simulink model "iface"  (R2018b)
settings: Solver=FixedStepDiscrete  StartTime=0.0  StopTime=10.0  RelTol=1e-3
settings Model: Creator=matlab  LastModifiedBy=matlab

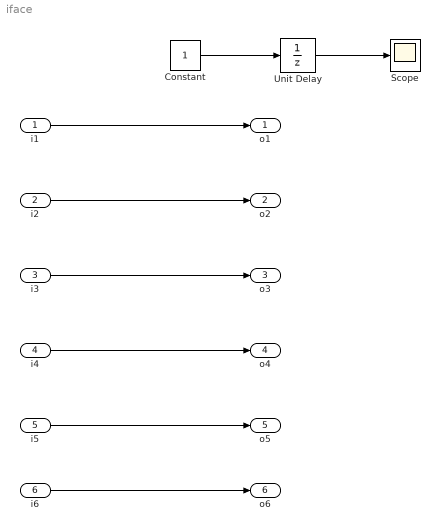
== system iface ==
  i1 : Inport  OutDataTypeStr=Enum: BoolSimulinkIntEnumType  PortDimensions=2
  i2 : Inport  Port=2  OutDataTypeStr=Enum: BoolUInt8Enum  PortDimensions=2
  i3 : Inport  Port=3  OutDataTypeStr=Enum: BoolUInt16Enum  PortDimensions=2
  i4 : Inport  Port=4  OutDataTypeStr=Enum: BoolInt8Enum  PortDimensions=2
  i5 : Inport  Port=5  OutDataTypeStr=Enum: BoolInt16Enum  PortDimensions=2
  i6 : Inport  Port=6  OutDataTypeStr=Enum: BoolInt32Enum  PortDimensions=2
  Constant : Constant
  Scope : Scope
  Unit Delay : UnitDelay  SampleTime=-1
  o1 : Outport  OutDataTypeStr=Enum: BoolSimulinkIntEnumType  PortDimensions=2
  o2 : Outport  Port=2  OutDataTypeStr=Enum: BoolUInt8Enum  PortDimensions=2
  o3 : Outport  Port=3  OutDataTypeStr=Enum: BoolUInt16Enum  PortDimensions=2
  o4 : Outport  Port=4  OutDataTypeStr=Enum: BoolInt8Enum  PortDimensions=2
  o5 : Outport  Port=5  OutDataTypeStr=Enum: BoolInt16Enum  PortDimensions=2
  o6 : Outport  Port=6  OutDataTypeStr=Enum: BoolInt32Enum  PortDimensions=2
  wires:
  i3/1 -> o3/1
  i2/1 -> o2/1
  i5/1 -> o5/1
  i6/1 -> o6/1
  i4/1 -> o4/1
  i1/1 -> o1/1
  Unit Delay/1 -> Scope/1
  Constant/1 -> Unit Delay/1
